simulink model "MultiReceive"  (Simulink 7.8)
settings: Solver=FixedStepDiscrete  SolverMode=SingleTasking  StartTime=0.0  StopTime=10.0  FixedStep=0.01  RelTol=1e-3
undefined symbols (not defined in the file): enqueueData, enqueueNumberText, Init_onlyOnce, Init_Reset, initCommunications, u1
libraries: dsPICdrivers x7, ecan_dspic x2, simulink x1
settings Model: Creator=Bryant  LastModifiedBy=Marx
settings OptimizationCC: InlineParams=on  OptimizeModelRefInitCode=on  LifeSpan=1
settings DebuggingCC: FcnCallInpInsideContextMsg=Use local settings
settings HardwareCC: ProdBitPerInt=16  ProdBitPerPointer=16  ProdEndianess=LittleEndian  ProdWordSize=16  ProdHWDeviceType=16-bit Generic
settings SFSimCC: SimParseCustomCode=off
settings RTWCC: SystemTargetFile=dspic.tlc  MakeCommand=make_CreateMPLAB  TemplateMakefile=dspic_pic30_gcc.tmf  PostCodeGenCommand=dsPIC_Compile()  Description=Embedded Target for Microchip dsPIC (real-time)  ProcessScript=dspic_make_rtw_hook
settings RTWCC: CustomSource=|
  | ../../CircularBuffer.c
  | ../../ecanFunctions.c
  | uart2.c
  | extra.c
settings CodeAppCC: IgnoreCustomStorageClasses=off
settings STFCustomTargetCC: IncludeMdlTerminateFcn=off  GeneratePreprocessorConditionals=Use local settings  CombineOutputUpdateFcns=on  SuppressErrorStatus=on  ERTCustomFileBanners=on  SupportContinuousTime=off  SupportNonInlinedSFcns=off  SystemTargetFile=dspic.tlc
settings ERTTargetCC: MultiwordLength=2048  ParMdlRefBuildCompliant=off  CompOptLevelCompliant=off  ConcurrentExecutionCompliant=off  IncludeMdlTerminateFcn=off  SuppressErrorStatus=on  ERTFirstTimeCompliant=off  ModelStepFunctionPrototypeControlCompliant=off  CPPClassGenCompliant=off  ExtModeMexFile=ext_serial_win32_comm  InlinedParameterPlacement=NonHierarchical  ERTSrcFileBannerTemplate=dsPIC_code_template.cgt  ERTHdrFileBannerTemplate=dsPIC_code_template.cgt  ERTDataSrcFileTemplate=dsPIC_code_template.cgt  ERTDataHdrFileTemplate=dsPIC_code_template.cgt  ERTCustomFileTemplate=dsPIC_main.tlc  ConvertIfToSwitch=off  SuppressUnreachableDefaultCases=off
settings CustomProperty: DataType=string  Value=C:\PROGRA~1\MATLAB\R2011b\bin\win64\gmake

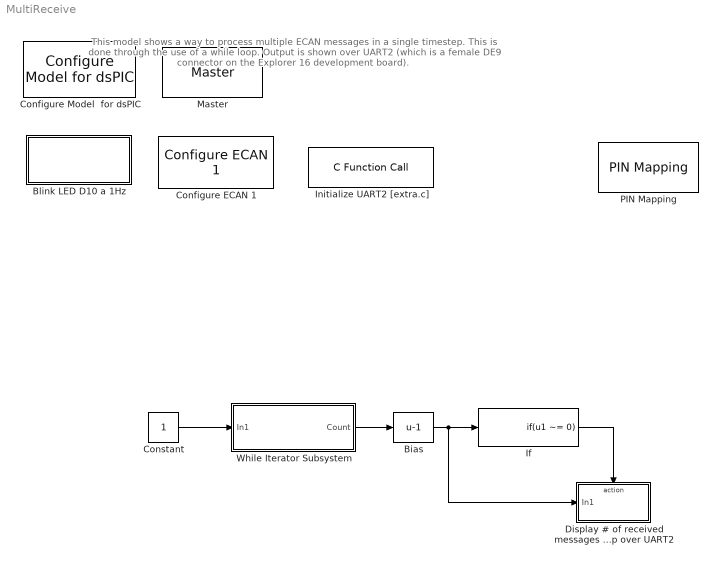
== system MultiReceive ==
  note: This model shows a way to process multiple ECAN messages in a single timestep. This is done through the use of a while loop.
      | Output is shown over UART2 (which is a female DE9 connector on the Explorer 16 development board).
  Bias : Bias  Bias=-1
  Blink LED D10 a 1Hz : Subsystem
      mask Display: disp('blink');
  Configure ECAN 1 : ecan_dspic/Configure ECAN 1  frame_setting=on  mode=Normal  dma_rx_chan=2  dma_tx_chan=0  baud=250000  ps1=8  pd=5  ps2=6  sjw=4  tq=20  triple_sample=on  dma_buf_size=4 buffers  rx_bufs=[1]  tx_bufs=[0]  buf_0_tx_pri=Highest  buf_0_rte=No  buf_1_tx_pri=Highest  buf_1_rte=No  buf_2_tx_pri=Lowest  buf_2_rte=No  buf_3_tx_pri=Lowest  buf_3_rte=No  buf_4_tx_pri=Lowest  buf_4_rte=No  buf_5_tx_pri=Lowest  buf_5_rte=No  buf_6_tx_pri=Lowest  buf_6_rte=No  buf_7_tx_pri=Lowest  buf_7_rte=No  mask_0=0  mask_0_mide=Match std or ext  mask_1=0  mask_1_mide=Match std or ext  mask_2=0  mask_2_mide=Match std or ext  filters=[0]  filter_0=0  filter_0_mask=0  filter_0_exide=Match only extended  filter_0_buf=1  filter_1=hex2dec('401')  filter_1_mask=0  filter_1_exide=Match only standard  filter_1_buf=2  filter_2=hex2dec('402')  filter_2_mask=0  filter_2_exide=Match only standard  filter_2_buf=3  filter_3=0  filter_3_mask=0  filter_3_exide=Match only standard  filter_3_buf=0  filter_4=0  filter_4_mask=0  filter_4_exide=Match only standard  filter_4_buf=0  filter_5=0  filter_5_mask=0  filter_5_exide=Match only standard  filter_5_buf=0  filter_6=0  filter_6_mask=0  filter_6_exide=Match only standard  filter_6_buf=0  filter_7=0  filter_7_mask=0  filter_7_exide=Match only standard  filter_7_buf=0  filter_8=0  filter_8_mask=0  filter_8_exide=Match only standard  filter_8_buf=0  filter_9=0  filter_9_mask=<empty>  filter_9_exide=Match only standard  filter_9_buf=0  filter_10=0  filter_10_mask=0  filter_10_exide=Match only standard  filter_10_buf=0  filter_11=0  filter_11_mask=0  filter_11_exide=Match only standard  filter_11_buf=0  filter_12=0  filter_12_mask=0  filter_12_exide=Match only standard  filter_12_buf=0  filter_13=0  filter_13_mask=0  filter_13_exide=Match only standard  filter_13_buf=0  filter_14=0  filter_14_mask=0  filter_14_exide=Match only standard  filter_14_buf=0  filter_15=0  filter_15_mask=0  filter_15_exide=Match only standard  filter_15_buf=0
  Configure Model  for dsPIC : dsPICdrivers/Simulink Configuration/Configure Model  for dsPIC
  Constant : Constant  SampleTime=.01
  Display # of received messages this timestep over UART2 : Subsystem  TreatAsAtomicUnit=on
  If : If  IfExpression=u1 ~= 0  ShowElse=off
  Initialize UART2 [extra.c] : dsPICdrivers/OTHERS/C Function Call  Tag=dsPIC_dsPIC_CFunctionCall  FctUpdate=None  fctName=enqueueNumberText  INPUT_SIZE=1  INPUT1=uint32  INPUT2=--  INPUT3=--  OUTPUT_SIZE=1  OUTPUT1=--  SampleTime=-1  InputType=[]  OutputType=[]  FctDeclaration=extern void enqueueNumberText();  FctCall=enqueueNumberText();  OrderingInOutPopup=None  FctStart=Start Function (Call once and only once)  FctStart_Name=initCommunications  FctStart_Declaration=inline extern void initCommunications();  FctStart_Call=initCommunications();  FctInit=None  FctInit_Name=Init_Reset  FctInit_Declaration=inline extern void Init_Reset();  FctInit_Call=Init_Reset();  PinDigitalInput=[]  PinDigitalOutput=[]  AnalogueInput=[]
  Master : dsPICdrivers/Master  Tag=dsPIC_MASTER  Priority=1  TimeStepType=Timer1  picType=33fj128MC802  fcy=40008571.4286  Quartz_33f=8e6  PLLActive_33f=on  fcyDesired_33f=40000000  tmr1="[8  50010  -0.00057131]"  tmr1Info="Time Step : 0.01  ;   Error : -0.00057131%  PR1=50010"  tmr2345="[0  0  0  0]"  tmr2345cfg=[-1 -1 -1 -1]  IOautoConf=on  typePort="[ 0   0   0   0  10   0   0   0   0   0   0   0   0   0   0   0   0   0   0   0  22  23  22  23   0   0   0   0   0   0   0   0   0   0   0   0   0   0   0   0   0   0   0   0   0   0   0   0   0   0   0   0   0   0   0   0   0   0   0   0   0   0   0   0   0   0   0   0   0   0   0   0   0   0   0   0   0   0   0   0   0   0   0   0   0   0   0   0   0   0   0   0   0   0   0   0   0   0   0   0   0   0   0   0   0   0   0   0   0   0   0   0 ]"  TRIS="[ 65519  65375  65535  65535  65535  65535  65535 ]"  ADPCFG=0  MasterBusyPort=None  MasterOverloadPort=None  FOSC=Internal Fast RC 7.37Mhz  ClockSwitchMonitor=Both disabled  TempProtection_33f=TEMP_ON  FPBOR=<empty>  PWRT=disable  MCLR=<empty>  ICD=ICS_PGD2  JTAGEN=JTAGEN_OFF  PowerSave=off  OverrideFcy=off  NewFcy=1e6  PR2345="[65535  65535  65535  65535]"
  PIN Mapping : dsPICdrivers/Peripheral MAPPING/PIN Mapping  Tag=dsPIC_PIN_Mapping  in_INT1=Not tied (VSS)  in_INT2=Not tied (VSS)  in_T2CK=Not tied (VSS)  in_T3CK=Not tied (VSS)  in_T4CK=Not tied (VSS)  in_T5CK=Not tied (VSS)  in_IC1=Not tied (VSS)  in_IC2=Not tied (VSS)  in_IC7=Not tied (VSS)  in_IC8=Not tied (VSS)  out_OC1=Not changed  out_OC2=Not changed  out_OC3=Not changed  out_OC4=Not changed  in_OCFA=Not tied (VSS)  in_FLTA1=Not tied (VSS)  in_FLTA2=Not tied (VSS)  in_QEA1=Not tied (VSS)  in_QEB1=Not tied (VSS)  in_INDX1=Not tied (VSS)  out_UPDN1=Not changed  out_UPDN2=Not changed  in_QEA2=Not tied (VSS)  in_QEB2=Not tied (VSS)  in_INDX2=Not tied (VSS)  in_U1RX=Not tied (VSS)  out_U1TX=Not changed  in_U1CTS=Not tied (VSS)  out_U1RTS=Not changed  in_U2RX=tied to RP4  out_U2TX=tied to RP5  in_U2CTS=Not tied (VSS)  out_U2RTS=Not changed  in_SDI1=Not tied (VSS)  out_SDO1=Not changed  in_SCK1=Not tied (VSS)  out_SCK1OUT=Not changed  in_SS1=Not tied (VSS)  out_SS1OUT=Not changed  in_SDI2=Not tied (VSS)  out_SDO2=Not changed  in_SCK2=Not tied (VSS)  out_SCK2OUT=Not changed  in_SS2=Not tied (VSS)  out_SS2OUT=Not changed  in_C1RX=tied to RP6  out_C1TX=tied to RP7  out_C1OUT=Not changed  out_C2OUT=Not changed
  While Iterator Subsystem : Subsystem  TreatAsAtomicUnit=on
  wires:
  While Iterator Subsystem/1(Count) -> Bias/1
  Constant/1 -> While Iterator Subsystem/1(In1)
  Bias/1 -> If/1, Display # of received messages this timestep over UART2/1(In1)
  If/1 -> Display # of received messages this timestep over UART2/Action

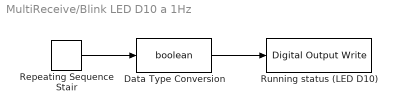
== system MultiReceive/Blink LED D10 a 1Hz ==
  Data Type Conversion : DataTypeConversion  OutDataTypeStr=boolean  RndMeth=Simplest
  Repeating Sequence Stair : simulink/Sources/Repeating Sequence Stair  OutValues=[1 0]  tsamp=1  OutMin=[]  OutMax=[]  OutDataTypeStr=double  OutputDataTypeScalingMode=double  OutDataType=fixdt(0,8)  ConRadixGroup=Best Precision: Vector-wise  OutScaling=2^-12
  Running status (LED D10) : dsPICdrivers/Digital I//O/Digital Output Write  Tag=dsPIC_Digital_Output  Priority=5  PORT=A  Pin=[4]  Simultaneous=off  OrderingInOutPopup=None
  wires:
  Repeating Sequence Stair/1 -> Data Type Conversion/1
  Data Type Conversion/1 -> Running status (LED D10)/1

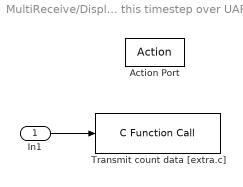
== system MultiReceive/Display # of received messages this timestep over UART2 ==
  In1 : Inport
  Action Port : ActionPort  ActionType=then
  Transmit count data [extra.c] : dsPICdrivers/OTHERS/C Function Call  Tag=dsPIC_dsPIC_CFunctionCall  FctUpdate=Output Function  fctName=enqueueData  INPUT_SIZE=1  INPUT1=int8  INPUT2=--  INPUT3=--  OUTPUT_SIZE=1  OUTPUT1=--  SampleTime=-1  InputType=[ 1 ]  OutputType=[ ]  FctDeclaration=extern void enqueueData(int8_T u1);  FctCall=enqueueData(%u1);  OrderingInOutPopup=None  FctStart=None  FctStart_Name=Init_onlyOnce  FctStart_Declaration=inline extern void Init_onlyOnce();  FctStart_Call=Init_onlyOnce();  FctInit=None  FctInit_Name=Init_Reset  FctInit_Declaration=inline extern void Init_Reset();  FctInit_Call=Init_Reset();  PinDigitalInput=[]  PinDigitalOutput=[]  AnalogueInput=[]
  wires:
  In1/1 -> Transmit count data [extra.c]/1

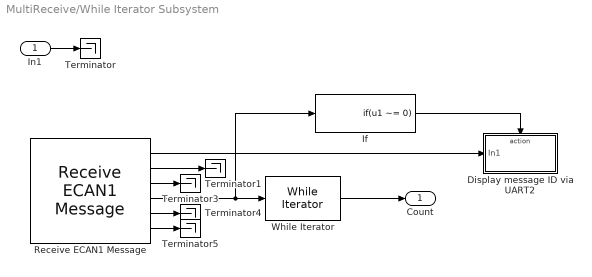
== system MultiReceive/While Iterator Subsystem ==
  In1 : Inport
  Display message ID via UART2 : Subsystem  TreatAsAtomicUnit=on
  If : If  IfExpression=u1 ~= 0  ShowElse=off
  Receive ECAN1 Message : ecan_dspic/Receive ECAN1 Message  ecan1_receive_sample_time=-1
  Terminator{,1,3..5} (5 alike) : Terminator
  While Iterator : WhileIterator  MaxIters=-1  WhileBlockType=do-while  ResetStates=reset  ShowIterationPort=on  OutputDataType=int8
  Count : Outport
  wires:
  Receive ECAN1 Message/4 -> While Iterator/1, If/1
  Receive ECAN1 Message/2 -> Terminator1/1
  Receive ECAN1 Message/3 -> Terminator3/1
  Receive ECAN1 Message/5 -> Terminator4/1
  While Iterator/1 -> Count/1
  Receive ECAN1 Message/6 -> Terminator5/1
  In1/1 -> Terminator/1
  Receive ECAN1 Message/1 -> Display message ID via UART2/1(In1)
  If/1 -> Display message ID via UART2/Action

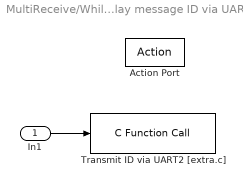
== system MultiReceive/While Iterator Subsystem/Display message ID via UART2 ==
  In1 : Inport
  Action Port : ActionPort  ActionType=then
  Transmit ID via UART2 [extra.c] : dsPICdrivers/OTHERS/C Function Call  Tag=dsPIC_dsPIC_CFunctionCall  FctUpdate=Output Function  fctName=enqueueNumberText  INPUT_SIZE=1  INPUT1=uint32  INPUT2=--  INPUT3=--  OUTPUT_SIZE=1  OUTPUT1=--  SampleTime=-1  InputType=[ 6 ]  OutputType=[ ]  FctDeclaration=extern void enqueueNumberText(uint32_T u1);  FctCall=enqueueNumberText(%u1);  OrderingInOutPopup=None  FctStart=None  FctStart_Name=Init_onlyOnce  FctStart_Declaration=inline extern void Init_onlyOnce();  FctStart_Call=Init_onlyOnce();  FctInit=None  FctInit_Name=Init_Reset  FctInit_Declaration=inline extern void Init_Reset();  FctInit_Call=Init_Reset();  PinDigitalInput=[]  PinDigitalOutput=[]  AnalogueInput=[]
  wires:
  In1/1 -> Transmit ID via UART2 [extra.c]/1
